simulink model "linear_double_track_model"  (R2023b)
settings: Solver=VariableStepAuto  StartTime=0.0  StopTime=10  RelTol=1e-3
undefined symbols (not defined in the file): cg_height, driver_mass, front_mass_distribution, static_toe_front, tire_loaded_radius, track_width_front, track_width_rear, vehicle_mass, wheelbase
libraries: autolibshared x1, vehdynlibsteering x1
settings Model: Creator=bglen  LastModifiedBy=bglen

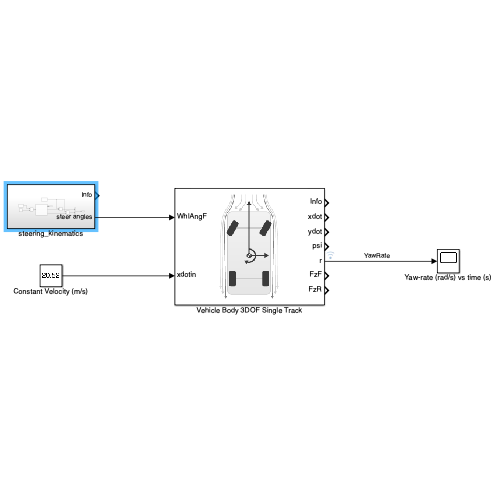
[thumbnail: Simulink's stored preview of the top-level diagram]
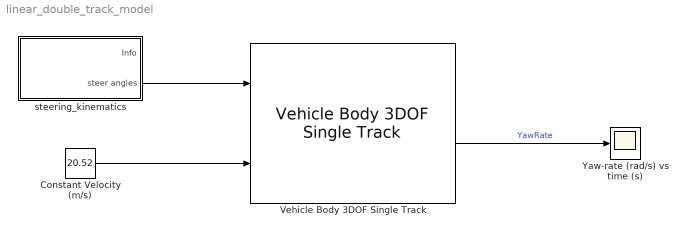
== system linear_double_track_model ==
  Constant Velocity (m/s) : Constant  Value=20.52
  Vehicle Body 3DOF Single Track : autolibshared/Vehicle Body 3DOF Single Track  trackMode=Dual  inputMode=External longitudinal velocity  frontSteerMode=on  rearSteerMode=off  windMode=off  muMode=off  extFMode=off  extMMode=off  htchFMode=off  htchMMode=off  extXo=off  extpsio=off  extxdoto=off  extro=off  extYo=off  extTamb=off  extydoto=off  aMode=2  NF=2  NR=2  m=vehicle_mass + driver_mass  a=wheelbase * (1 - front_mass_distribution)  b=wheelbase * front_mass_distribution  h=cg_height - tire_loaded_radius  dh=1  hh=0.2  X_o=0  xdot_o=0  CalphaMode=off  sigmaMode=off  d=0  hl=0  w=[track_width_front,track_width_rear]  Cy_f=28648  Cy_r=28648  sigma_f=.1  sigma_r=.1  alpha_f_brk=[-.1 .1]  Cy_f_data=[-9e3 9e3]  alpha_r_brk=[-.1 .1]  Cy_r_data=[-9e3 9e3]  Y_o=0  ydot_o=0  Izz=yaw_polar_inertia  psi_o=0  r_o=0  Af=frontal_area  Cd=Cd  Cl=Cl  Cpm=0  beta_w=[0 0.01:0.01:0.3]  Cs=[0 0.01:0.01:0.3]  Cym=[0 1e-6:0.01:0.3]  Pabs=101325  Tair=273  g=9.81  mu=1  xdot_tol=.01  Fznom=(vehicle_mass + driver_mass) * 9.81  Fxtire_sat=7e4  Fytire_sat=7e4  longOff=0  latOff=0  vertOff=0  wrapAng=off
  Yaw-rate (rad/s) vs time (s) : Scope
  steering_kinematics : Subsystem
  wires:
  Constant Velocity (m/s)/1 -> Vehicle Body 3DOF Single Track/2
  Vehicle Body 3DOF Single Track/5 -> Yaw-rate (rad/s) vs time (s)/1  "YawRate"
  steering_kinematics/2(steer angles) -> Vehicle Body 3DOF Single Track/1

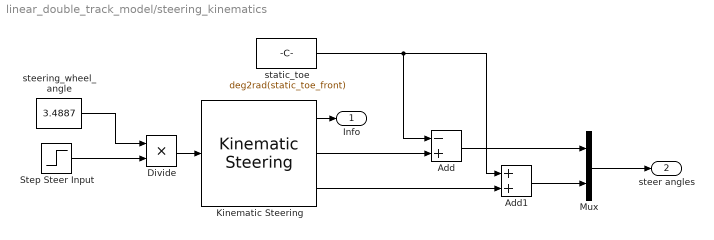
== system linear_double_track_model/steering_kinematics ==
  Add : Sum  Inputs=-+
  Add1 : Sum
  Divide : Product  Inputs=**
  Kinematic Steering : vehdynlibsteering/Kinematic Steering  StrgType=Ackerman  StrgRatioType=Constant  Loc=Front  NrmlFctr=1  TrckWdth=track_width_front  WhlBase=wheelbase  Db=0  StrgRng=pi  StrgAngBpts="[-6.2832   -5.0265   -3.7699   -2.5133   -1.2566         0    1.2566    2.5133    3.7699    5.0265    6.2832]"  StrgRatioTbl=|  StrgRatio=steering_ratio  PctAckIn=off  PctAck=ackerman_percentage  PctAckTbl=ones(1,11)*100  StrgArmLngth=0.1  RckCsLngth=0.5  TieRodLngth=0.248  D=0.2  PnnRadius=0.00085818  PnnRadiusTbl="[0.0055    0.0055    0.0056    0.0057    0.0058    0.0057    0.0057    0.0057    0.0056    0.0055    0.0055]"  RodLngth=0.1  ParaArmLngth=0.9  aMode=2
      | [13.5000   13.3750   13.2500   13.1250   13.0000   13.0000   13.0000   13.1250   13.2500   13.3750   13.5000
      | ]
  Mux : Mux  Inputs=2
  Step Steer Input : Step  SampleTime=0
  static_toe : Constant  Value=deg2rad(static_toe_front)
  steering_wheel_angle : Constant  Value=3.4887
  Info : Outport
  steer angles : Outport  Port=2
  wires:
  Add1/1 -> Mux/2
  Mux/1 -> steer angles/1
  Kinematic Steering/2 -> Add/2
  static_toe/1 -> Add/1, Add1/1
  Kinematic Steering/1 -> Info/1
  Add/1 -> Mux/1
  Kinematic Steering/3 -> Add1/2
  Divide/1 -> Kinematic Steering/1
  Step Steer Input/1 -> Divide/2
  steering_wheel_angle/1 -> Divide/1
